simulink model "station_no_recovery"  (R2015a)
settings: Solver=ode45  StartTime=0  StopTime=5000  FixedStep=10  MaxStep=1  RelTol=1e-3
(part 3 of 4)

== system station_no_recovery/Восстанавливаемые объекты/САТУРН/Subsystem2 ==
  λ1 : Inport
  λ2 : Inport  Port=2
  M : Inport  Port=3
  dP : Inport  Port=4
  Pz : Inport  Port=5
  dt : Inport  Port=6
  trec : Inport  Port=7
  t_start : Inport  Port=8
  Chart : Stateflow chart  TreatAsAtomicUnit=on
  Clock : Clock
  Data Store Memory : DataStoreMemory  DataStoreName=t3_3
  Data Store Read : DataStoreRead  DataStoreName=t3_3
  Data Store Write : DataStoreWrite  DataStoreName=t3_3
  Element Exponential : Subsystem  mask(Element Exponential){}
      mask help:
      | <p>Возвращает вероятность безотказной работы невосстанавливаемого элемента
      | по экспоненциальному закону распределения.</p>
      | <p>Экспоненциальное (или показательное) распределение — абсолютно непрерывное
      | распределение, моделирующее время между двумя последовательными свершениями
      | одного и того же события.</p>
      | <p>Экспоненциальное распределение используют при оценке надежности сложных
      | технических систем, не подверженных износу и старению и в случаях, когда
      | отказы объектов имеют случайный характер.</p>
      mask Help:
      | <p>Возвращает вероятность безотказной работы невосстанавливаемого элемента по экспоненциальному
      | закону распределения.</p>
      | <p>Экспоненциальное распределение используют при оценке надежности сложных
      | технических систем, не подверженных износу и старению и в случаях, когда
      | отказы объектов имеют случайный характер.</p>
      | <p>Входной параметр λ - интенсивность событий в рассматриваемом потоке.</p>
      | <p>Выходной параметр P(t) - вероятность безотказной работы элемента.</p>
      mask Display:
      | image('images/png/exp.png')
      | port_label('input', 1, 'λ')
      | port_label('output', 1, 'P(t)')
  Element Normal : Subsystem  mask(Element Normal){}
      mask help:
      | <p>Возвращает вероятность безотказной работы невосстанавливаемого
      | элемента по нормальному закону распределения.</p>
      | <p>Нормальное распределение, также называемое распределением Гаусса или
      | Гаусса — Лапласа — распределение вероятностей, которое в одномерном
      | случае задаётся функцией плотности вероятности, совпадающей с функцией
      | Гаусса.</p>
      | <p>Нормальное распределение обычно используют при оценке надежности объектов,
      | основной причиной отказа которых является износ.</p>
      mask Help:
      | <p>Возвращает вероятность безотказной работы невосстанавливаемого
      | элемента по нормальному закону распределения.</p>
      | <p>Нормальное распределение обычно используют при оценке надежности объектов,
      | основной причиной отказа которых является износ.</p>
      | <p>Входные параметры:</p>
      | <p>λ - среднее квадратическое отклонение наработки до отказа,</p>
      | <p>М - математическое ожидание наработки до отказа.</p>
      | <p>Выходной параметр P(t) - вероятность безотказной работы элемента.</p>
      mask Display:
      | image('images/png/normal_nogrid.png')
      | port_label('input', 1, 'λ')
      | port_label('input', 2, 'M')
      | port_label('output', 1, 'P(t)')
  Сircuit Series : Subsystem  mask(Сircuit Series){}
      mask help:
      | <p>Возвращает вероятность безотказной работы двух последовательно соединенных
      | элементов.</p>
      | <p>В системе с последовательной структурой отказ любого компонента приводит
      | к отказу системы в целом.</p>
      mask Help:
      | <p>Возвращает вероятность безотказной работы двух последовательно соединенных
      | элементов.</p>
      | <p>Входные параметры:</p>
      | <p>P1 - вероятность безотказной работы первого элемента,</p>
      | <p>P2 - вероятность безотказной работы второго элемента.</p>
      | <p>Выходной параметр P12 - вероятность безотказной работы двух последовательно
      | соединенных элементов.</p>
      mask Display:
      | image('images/png/series2.png')
      | port_label('input', 1, 'P1')
      | port_label('input', 2, 'P2')
      | port_label('output', 1, 'P12')
  P : Outport
  wires:
  Element Exponential/1(P(t)1) -> Сircuit Series/1(P1)
  Element Normal/1(P(t)) -> Сircuit Series/2(P2)
  Chart/2(P) -> P/1
  λ2/1 -> Element Normal/1("lambda ")
  Clock/1 -> Chart/6(t)
  Сircuit Series/1(P12) -> Chart/7(P0)
  dt/1 -> Chart/2(delta_t)
  λ1/1 -> Element Exponential/1("lambda ")
  Pz/1 -> Chart/3(Pz)
  dP/1 -> Chart/5(dP)
  M/1 -> Element Normal/2("M ")
  trec/1 -> Chart/4(trec)
  Data Store Read/1 -> Element Exponential/2(t), Element Normal/3(t)
  Chart/1(tv) -> Data Store Write/1
  t_start/1 -> Chart/1(t_start)

== system station_no_recovery/Восстанавливаемые объекты/САТУРН/Subsystem3 ==
  λ1 : Inport
  λ2 : Inport  Port=2
  M : Inport  Port=3
  dP : Inport  Port=4
  Pz : Inport  Port=5
  dt : Inport  Port=6
  trec : Inport  Port=7
  t_start : Inport  Port=8
  Chart : Stateflow chart  TreatAsAtomicUnit=on
  Clock : Clock
  Data Store Memory : DataStoreMemory  DataStoreName=t3_4
  Data Store Read : DataStoreRead  DataStoreName=t3_4
  Data Store Write : DataStoreWrite  DataStoreName=t3_4
  Element Exponential : Subsystem  mask(Element Exponential){}
      mask help:
      | <p>Возвращает вероятность безотказной работы невосстанавливаемого элемента
      | по экспоненциальному закону распределения.</p>
      | <p>Экспоненциальное (или показательное) распределение — абсолютно непрерывное
      | распределение, моделирующее время между двумя последовательными свершениями
      | одного и того же события.</p>
      | <p>Экспоненциальное распределение используют при оценке надежности сложных
      | технических систем, не подверженных износу и старению и в случаях, когда
      | отказы объектов имеют случайный характер.</p>
      mask Help:
      | <p>Возвращает вероятность безотказной работы невосстанавливаемого элемента по экспоненциальному
      | закону распределения.</p>
      | <p>Экспоненциальное распределение используют при оценке надежности сложных
      | технических систем, не подверженных износу и старению и в случаях, когда
      | отказы объектов имеют случайный характер.</p>
      | <p>Входной параметр λ - интенсивность событий в рассматриваемом потоке.</p>
      | <p>Выходной параметр P(t) - вероятность безотказной работы элемента.</p>
      mask Display:
      | image('images/png/exp.png')
      | port_label('input', 1, 'λ')
      | port_label('output', 1, 'P(t)')
  Element Normal : Subsystem  mask(Element Normal){}
      mask help:
      | <p>Возвращает вероятность безотказной работы невосстанавливаемого
      | элемента по нормальному закону распределения.</p>
      | <p>Нормальное распределение, также называемое распределением Гаусса или
      | Гаусса — Лапласа — распределение вероятностей, которое в одномерном
      | случае задаётся функцией плотности вероятности, совпадающей с функцией
      | Гаусса.</p>
      | <p>Нормальное распределение обычно используют при оценке надежности объектов,
      | основной причиной отказа которых является износ.</p>
      mask Help:
      | <p>Возвращает вероятность безотказной работы невосстанавливаемого
      | элемента по нормальному закону распределения.</p>
      | <p>Нормальное распределение обычно используют при оценке надежности объектов,
      | основной причиной отказа которых является износ.</p>
      | <p>Входные параметры:</p>
      | <p>λ - среднее квадратическое отклонение наработки до отказа,</p>
      | <p>М - математическое ожидание наработки до отказа.</p>
      | <p>Выходной параметр P(t) - вероятность безотказной работы элемента.</p>
      mask Display:
      | image('images/png/normal_nogrid.png')
      | port_label('input', 1, 'λ')
      | port_label('input', 2, 'M')
      | port_label('output', 1, 'P(t)')
  Сircuit Series : Subsystem  mask(Сircuit Series){}
      mask help:
      | <p>Возвращает вероятность безотказной работы двух последовательно соединенных
      | элементов.</p>
      | <p>В системе с последовательной структурой отказ любого компонента приводит
      | к отказу системы в целом.</p>
      mask Help:
      | <p>Возвращает вероятность безотказной работы двух последовательно соединенных
      | элементов.</p>
      | <p>Входные параметры:</p>
      | <p>P1 - вероятность безотказной работы первого элемента,</p>
      | <p>P2 - вероятность безотказной работы второго элемента.</p>
      | <p>Выходной параметр P12 - вероятность безотказной работы двух последовательно
      | соединенных элементов.</p>
      mask Display:
      | image('images/png/series2.png')
      | port_label('input', 1, 'P1')
      | port_label('input', 2, 'P2')
      | port_label('output', 1, 'P12')
  P : Outport
  wires:
  t_start/1 -> Chart/1(t_start)
  Chart/1(tv) -> Data Store Write/1
  Data Store Read/1 -> Element Normal/3(t), Element Exponential/2(t)
  trec/1 -> Chart/4(trec)
  M/1 -> Element Normal/2("M ")
  dP/1 -> Chart/5(dP)
  Pz/1 -> Chart/3(Pz)
  λ1/1 -> Element Exponential/1("lambda ")
  dt/1 -> Chart/2(delta_t)
  Сircuit Series/1(P12) -> Chart/7(P0)
  Clock/1 -> Chart/6(t)
  λ2/1 -> Element Normal/1("lambda ")
  Chart/2(P) -> P/1
  Element Normal/1(P(t)) -> Сircuit Series/2(P2)
  Element Exponential/1(P(t)1) -> Сircuit Series/1(P1)

== system station_no_recovery/Восстанавливаемые объекты/САТУРН/Subsystem4 ==
  λ1 : Inport
  λ2 : Inport  Port=2
  M : Inport  Port=3
  dP : Inport  Port=4
  Pz : Inport  Port=5
  dt : Inport  Port=6
  trec : Inport  Port=7
  t_start : Inport  Port=8
  Chart : Stateflow chart  TreatAsAtomicUnit=on
  Clock : Clock
  Data Store Memory : DataStoreMemory  DataStoreName=t3_1
  Data Store Read : DataStoreRead  DataStoreName=t3_1
  Data Store Write : DataStoreWrite  DataStoreName=t3_1
  Element Exponential : Subsystem  mask(Element Exponential){}
      mask help:
      | <p>Возвращает вероятность безотказной работы невосстанавливаемого элемента
      | по экспоненциальному закону распределения.</p>
      | <p>Экспоненциальное (или показательное) распределение — абсолютно непрерывное
      | распределение, моделирующее время между двумя последовательными свершениями
      | одного и того же события.</p>
      | <p>Экспоненциальное распределение используют при оценке надежности сложных
      | технических систем, не подверженных износу и старению и в случаях, когда
      | отказы объектов имеют случайный характер.</p>
      mask Help:
      | <p>Возвращает вероятность безотказной работы невосстанавливаемого элемента по экспоненциальному
      | закону распределения.</p>
      | <p>Экспоненциальное распределение используют при оценке надежности сложных
      | технических систем, не подверженных износу и старению и в случаях, когда
      | отказы объектов имеют случайный характер.</p>
      | <p>Входной параметр λ - интенсивность событий в рассматриваемом потоке.</p>
      | <p>Выходной параметр P(t) - вероятность безотказной работы элемента.</p>
      mask Display:
      | image('images/png/exp.png')
      | port_label('input', 1, 'λ')
      | port_label('output', 1, 'P(t)')
  Element Normal : Subsystem  mask(Element Normal){}
      mask help:
      | <p>Возвращает вероятность безотказной работы невосстанавливаемого
      | элемента по нормальному закону распределения.</p>
      | <p>Нормальное распределение, также называемое распределением Гаусса или
      | Гаусса — Лапласа — распределение вероятностей, которое в одномерном
      | случае задаётся функцией плотности вероятности, совпадающей с функцией
      | Гаусса.</p>
      | <p>Нормальное распределение обычно используют при оценке надежности объектов,
      | основной причиной отказа которых является износ.</p>
      mask Help:
      | <p>Возвращает вероятность безотказной работы невосстанавливаемого
      | элемента по нормальному закону распределения.</p>
      | <p>Нормальное распределение обычно используют при оценке надежности объектов,
      | основной причиной отказа которых является износ.</p>
      | <p>Входные параметры:</p>
      | <p>λ - среднее квадратическое отклонение наработки до отказа,</p>
      | <p>М - математическое ожидание наработки до отказа.</p>
      | <p>Выходной параметр P(t) - вероятность безотказной работы элемента.</p>
      mask Display:
      | image('images/png/normal_nogrid.png')
      | port_label('input', 1, 'λ')
      | port_label('input', 2, 'M')
      | port_label('output', 1, 'P(t)')
  Сircuit Series : Subsystem  mask(Сircuit Series){}
      mask help:
      | <p>Возвращает вероятность безотказной работы двух последовательно соединенных
      | элементов.</p>
      | <p>В системе с последовательной структурой отказ любого компонента приводит
      | к отказу системы в целом.</p>
      mask Help:
      | <p>Возвращает вероятность безотказной работы двух последовательно соединенных
      | элементов.</p>
      | <p>Входные параметры:</p>
      | <p>P1 - вероятность безотказной работы первого элемента,</p>
      | <p>P2 - вероятность безотказной работы второго элемента.</p>
      | <p>Выходной параметр P12 - вероятность безотказной работы двух последовательно
      | соединенных элементов.</p>
      mask Display:
      | image('images/png/series2.png')
      | port_label('input', 1, 'P1')
      | port_label('input', 2, 'P2')
      | port_label('output', 1, 'P12')
  P : Outport
  wires:
  Element Exponential/1(P(t)1) -> Сircuit Series/1(P1)
  Element Normal/1(P(t)) -> Сircuit Series/2(P2)
  Chart/2(P) -> P/1
  λ2/1 -> Element Normal/1("lambda ")
  Clock/1 -> Chart/6(t)
  Сircuit Series/1(P12) -> Chart/7(P0)
  dt/1 -> Chart/2(delta_t)
  λ1/1 -> Element Exponential/1("lambda ")
  Pz/1 -> Chart/3(Pz)
  dP/1 -> Chart/5(dP)
  M/1 -> Element Normal/2("M ")
  trec/1 -> Chart/4(trec)
  Data Store Read/1 -> Element Exponential/2(t), Element Normal/3(t)
  Chart/1(tv) -> Data Store Write/1
  t_start/1 -> Chart/1(t_start)

== system station_no_recovery/Восстанавливаемые объекты/УРАЛ-6000/Subsystem1 ==
  λ1 : Inport
  λ2 : Inport  Port=2
  M : Inport  Port=3
  dP : Inport  Port=4
  Pz : Inport  Port=5
  dt : Inport  Port=6
  trec : Inport  Port=7
  t_start : Inport  Port=8
  Chart : Stateflow chart  TreatAsAtomicUnit=on
  Clock : Clock
  Data Store Memory : DataStoreMemory  DataStoreName=t2_2
  Data Store Read : DataStoreRead  DataStoreName=t2_2
  Data Store Write : DataStoreWrite  DataStoreName=t2_2
  Display : Display
  Element Exponential : Subsystem  mask(Element Exponential){}
      mask help:
      | <p>Возвращает вероятность безотказной работы невосстанавливаемого элемента
      | по экспоненциальному закону распределения.</p>
      | <p>Экспоненциальное (или показательное) распределение — абсолютно непрерывное
      | распределение, моделирующее время между двумя последовательными свершениями
      | одного и того же события.</p>
      | <p>Экспоненциальное распределение используют при оценке надежности сложных
      | технических систем, не подверженных износу и старению и в случаях, когда
      | отказы объектов имеют случайный характер.</p>
      mask Help:
      | <p>Возвращает вероятность безотказной работы невосстанавливаемого элемента по экспоненциальному
      | закону распределения.</p>
      | <p>Экспоненциальное распределение используют при оценке надежности сложных
      | технических систем, не подверженных износу и старению и в случаях, когда
      | отказы объектов имеют случайный характер.</p>
      | <p>Входной параметр λ - интенсивность событий в рассматриваемом потоке.</p>
      | <p>Выходной параметр P(t) - вероятность безотказной работы элемента.</p>
      mask Display:
      | image('images/png/exp.png')
      | port_label('input', 1, 'λ')
      | port_label('output', 1, 'P(t)')
  Element Normal : Subsystem  mask(Element Normal){}
      mask help:
      | <p>Возвращает вероятность безотказной работы невосстанавливаемого
      | элемента по нормальному закону распределения.</p>
      | <p>Нормальное распределение, также называемое распределением Гаусса или
      | Гаусса — Лапласа — распределение вероятностей, которое в одномерном
      | случае задаётся функцией плотности вероятности, совпадающей с функцией
      | Гаусса.</p>
      | <p>Нормальное распределение обычно используют при оценке надежности объектов,
      | основной причиной отказа которых является износ.</p>
      mask Help:
      | <p>Возвращает вероятность безотказной работы невосстанавливаемого
      | элемента по нормальному закону распределения.</p>
      | <p>Нормальное распределение обычно используют при оценке надежности объектов,
      | основной причиной отказа которых является износ.</p>
      | <p>Входные параметры:</p>
      | <p>λ - среднее квадратическое отклонение наработки до отказа,</p>
      | <p>М - математическое ожидание наработки до отказа.</p>
      | <p>Выходной параметр P(t) - вероятность безотказной работы элемента.</p>
      mask Display:
      | image('images/png/normal_nogrid.png')
      | port_label('input', 1, 'λ')
      | port_label('input', 2, 'M')
      | port_label('output', 1, 'P(t)')
  Mux : Mux  Inputs=2
  Сircuit Series : Subsystem  mask(Сircuit Series){}
      mask help:
      | <p>Возвращает вероятность безотказной работы двух последовательно соединенных
      | элементов.</p>
      | <p>В системе с последовательной структурой отказ любого компонента приводит
      | к отказу системы в целом.</p>
      mask Help:
      | <p>Возвращает вероятность безотказной работы двух последовательно соединенных
      | элементов.</p>
      | <p>Входные параметры:</p>
      | <p>P1 - вероятность безотказной работы первого элемента,</p>
      | <p>P2 - вероятность безотказной работы второго элемента.</p>
      | <p>Выходной параметр P12 - вероятность безотказной работы двух последовательно
      | соединенных элементов.</p>
      mask Display:
      | image('images/png/series2.png')
      | port_label('input', 1, 'P1')
      | port_label('input', 2, 'P2')
      | port_label('output', 1, 'P12')
  P : Outport
  wires:
  Data Store Read/1 -> Element Exponential/2(t), Mux/2, Element Normal/3(t)
  t_start/1 -> Chart/1(t_start)
  Chart/1(tv) -> Data Store Write/1
  Mux/1 -> Display/1
  Сircuit Series/1(P12) -> Chart/7(P0)
  trec/1 -> Chart/4(trec)
  M/1 -> Element Normal/2("M ")
  dP/1 -> Chart/5(dP)
  Pz/1 -> Chart/3(Pz)
  λ1/1 -> Element Exponential/1("lambda "), Mux/1
  dt/1 -> Chart/2(delta_t)
  Clock/1 -> Chart/6(t)
  λ2/1 -> Element Normal/1("lambda ")
  Chart/2(P) -> P/1
  Element Normal/1(P(t)) -> Сircuit Series/2(P2)
  Element Exponential/1(P(t)1) -> Сircuit Series/1(P1)

== system station_no_recovery/Восстанавливаемые объекты/УРАЛ-6000/Subsystem2 ==
  λ1 : Inport
  λ2 : Inport  Port=2
  M : Inport  Port=3
  dP : Inport  Port=4
  Pz : Inport  Port=5
  dt : Inport  Port=6
  trec : Inport  Port=7
  t_start : Inport  Port=8
  Chart : Stateflow chart  TreatAsAtomicUnit=on
  Clock : Clock
  Data Store Memory : DataStoreMemory  DataStoreName=t2_1
  Data Store Read : DataStoreRead  DataStoreName=t2_1
  Data Store Write : DataStoreWrite  DataStoreName=t2_1
  Display : Display
  Element Exponential : Subsystem  mask(Element Exponential){}
      mask help:
      | <p>Возвращает вероятность безотказной работы невосстанавливаемого элемента
      | по экспоненциальному закону распределения.</p>
      | <p>Экспоненциальное (или показательное) распределение — абсолютно непрерывное
      | распределение, моделирующее время между двумя последовательными свершениями
      | одного и того же события.</p>
      | <p>Экспоненциальное распределение используют при оценке надежности сложных
      | технических систем, не подверженных износу и старению и в случаях, когда
      | отказы объектов имеют случайный характер.</p>
      mask Help:
      | <p>Возвращает вероятность безотказной работы невосстанавливаемого элемента по экспоненциальному
      | закону распределения.</p>
      | <p>Экспоненциальное распределение используют при оценке надежности сложных
      | технических систем, не подверженных износу и старению и в случаях, когда
      | отказы объектов имеют случайный характер.</p>
      | <p>Входной параметр λ - интенсивность событий в рассматриваемом потоке.</p>
      | <p>Выходной параметр P(t) - вероятность безотказной работы элемента.</p>
      mask Display:
      | image('images/png/exp.png')
      | port_label('input', 1, 'λ')
      | port_label('output', 1, 'P(t)')
  Element Normal : Subsystem  mask(Element Normal){}
      mask help:
      | <p>Возвращает вероятность безотказной работы невосстанавливаемого
      | элемента по нормальному закону распределения.</p>
      | <p>Нормальное распределение, также называемое распределением Гаусса или
      | Гаусса — Лапласа — распределение вероятностей, которое в одномерном
      | случае задаётся функцией плотности вероятности, совпадающей с функцией
      | Гаусса.</p>
      | <p>Нормальное распределение обычно используют при оценке надежности объектов,
      | основной причиной отказа которых является износ.</p>
      mask Help:
      | <p>Возвращает вероятность безотказной работы невосстанавливаемого
      | элемента по нормальному закону распределения.</p>
      | <p>Нормальное распределение обычно используют при оценке надежности объектов,
      | основной причиной отказа которых является износ.</p>
      | <p>Входные параметры:</p>
      | <p>λ - среднее квадратическое отклонение наработки до отказа,</p>
      | <p>М - математическое ожидание наработки до отказа.</p>
      | <p>Выходной параметр P(t) - вероятность безотказной работы элемента.</p>
      mask Display:
      | image('images/png/normal_nogrid.png')
      | port_label('input', 1, 'λ')
      | port_label('input', 2, 'M')
      | port_label('output', 1, 'P(t)')
  Mux : Mux  Inputs=2
  Сircuit Series : Subsystem  mask(Сircuit Series){}
      mask help:
      | <p>Возвращает вероятность безотказной работы двух последовательно соединенных
      | элементов.</p>
      | <p>В системе с последовательной структурой отказ любого компонента приводит
      | к отказу системы в целом.</p>
      mask Help:
      | <p>Возвращает вероятность безотказной работы двух последовательно соединенных
      | элементов.</p>
      | <p>Входные параметры:</p>
      | <p>P1 - вероятность безотказной работы первого элемента,</p>
      | <p>P2 - вероятность безотказной работы второго элемента.</p>
      | <p>Выходной параметр P12 - вероятность безотказной работы двух последовательно
      | соединенных элементов.</p>
      mask Display:
      | image('images/png/series2.png')
      | port_label('input', 1, 'P1')
      | port_label('input', 2, 'P2')
      | port_label('output', 1, 'P12')
  P : Outport
  wires:
  Element Exponential/1(P(t)1) -> Сircuit Series/1(P1)
  Element Normal/1(P(t)) -> Сircuit Series/2(P2)
  Chart/2(P) -> P/1
  λ2/1 -> Element Normal/1("lambda ")
  Clock/1 -> Chart/6(t)
  dt/1 -> Chart/2(delta_t)
  λ1/1 -> Mux/1, Element Exponential/1("lambda ")
  Pz/1 -> Chart/3(Pz)
  dP/1 -> Chart/5(dP)
  M/1 -> Element Normal/2("M ")
  trec/1 -> Chart/4(trec)
  Сircuit Series/1(P12) -> Chart/7(P0)
  Mux/1 -> Display/1
  Chart/1(tv) -> Data Store Write/1
  t_start/1 -> Chart/1(t_start)
  Data Store Read/1 -> Element Normal/3(t), Mux/2, Element Exponential/2(t)

== system station_no_recovery/Восстанавливаемые объекты/УРАЛ-6000/Subsystem3 ==
  λ1 : Inport
  λ2 : Inport  Port=2
  M : Inport  Port=3
  dP : Inport  Port=4
  Pz : Inport  Port=5
  dt : Inport  Port=6
  trec : Inport  Port=7
  t_start : Inport  Port=8
  Chart : Stateflow chart  TreatAsAtomicUnit=on
  Clock : Clock
  Data Store Memory : DataStoreMemory  DataStoreName=t2_3
  Data Store Read : DataStoreRead  DataStoreName=t2_3
  Data Store Write : DataStoreWrite  DataStoreName=t2_3
  Display : Display
  Element Exponential : Subsystem  mask(Element Exponential){}
      mask help:
      | <p>Возвращает вероятность безотказной работы невосстанавливаемого элемента
      | по экспоненциальному закону распределения.</p>
      | <p>Экспоненциальное (или показательное) распределение — абсолютно непрерывное
      | распределение, моделирующее время между двумя последовательными свершениями
      | одного и того же события.</p>
      | <p>Экспоненциальное распределение используют при оценке надежности сложных
      | технических систем, не подверженных износу и старению и в случаях, когда
      | отказы объектов имеют случайный характер.</p>
      mask Help:
      | <p>Возвращает вероятность безотказной работы невосстанавливаемого элемента по экспоненциальному
      | закону распределения.</p>
      | <p>Экспоненциальное распределение используют при оценке надежности сложных
      | технических систем, не подверженных износу и старению и в случаях, когда
      | отказы объектов имеют случайный характер.</p>
      | <p>Входной параметр λ - интенсивность событий в рассматриваемом потоке.</p>
      | <p>Выходной параметр P(t) - вероятность безотказной работы элемента.</p>
      mask Display:
      | image('images/png/exp.png')
      | port_label('input', 1, 'λ')
      | port_label('output', 1, 'P(t)')
  Element Normal : Subsystem  mask(Element Normal){}
      mask help:
      | <p>Возвращает вероятность безотказной работы невосстанавливаемого
      | элемента по нормальному закону распределения.</p>
      | <p>Нормальное распределение, также называемое распределением Гаусса или
      | Гаусса — Лапласа — распределение вероятностей, которое в одномерном
      | случае задаётся функцией плотности вероятности, совпадающей с функцией
      | Гаусса.</p>
      | <p>Нормальное распределение обычно используют при оценке надежности объектов,
      | основной причиной отказа которых является износ.</p>
      mask Help:
      | <p>Возвращает вероятность безотказной работы невосстанавливаемого
      | элемента по нормальному закону распределения.</p>
      | <p>Нормальное распределение обычно используют при оценке надежности объектов,
      | основной причиной отказа которых является износ.</p>
      | <p>Входные параметры:</p>
      | <p>λ - среднее квадратическое отклонение наработки до отказа,</p>
      | <p>М - математическое ожидание наработки до отказа.</p>
      | <p>Выходной параметр P(t) - вероятность безотказной работы элемента.</p>
      mask Display:
      | image('images/png/normal_nogrid.png')
      | port_label('input', 1, 'λ')
      | port_label('input', 2, 'M')
      | port_label('output', 1, 'P(t)')
  Mux : Mux  Inputs=2
  Сircuit Series : Subsystem  mask(Сircuit Series){}
      mask help:
      | <p>Возвращает вероятность безотказной работы двух последовательно соединенных
      | элементов.</p>
      | <p>В системе с последовательной структурой отказ любого компонента приводит
      | к отказу системы в целом.</p>
      mask Help:
      | <p>Возвращает вероятность безотказной работы двух последовательно соединенных
      | элементов.</p>
      | <p>Входные параметры:</p>
      | <p>P1 - вероятность безотказной работы первого элемента,</p>
      | <p>P2 - вероятность безотказной работы второго элемента.</p>
      | <p>Выходной параметр P12 - вероятность безотказной работы двух последовательно
      | соединенных элементов.</p>
      mask Display:
      | image('images/png/series2.png')
      | port_label('input', 1, 'P1')
      | port_label('input', 2, 'P2')
      | port_label('output', 1, 'P12')
  P : Outport
  wires:
  Element Exponential/1(P(t)1) -> Сircuit Series/1(P1)
  Element Normal/1(P(t)) -> Сircuit Series/2(P2)
  Chart/2(P) -> P/1
  λ2/1 -> Element Normal/1("lambda ")
  Clock/1 -> Chart/6(t)
  dt/1 -> Chart/2(delta_t)
  λ1/1 -> Mux/1, Element Exponential/1("lambda ")
  Pz/1 -> Chart/3(Pz)
  dP/1 -> Chart/5(dP)
  M/1 -> Element Normal/2("M ")
  trec/1 -> Chart/4(trec)
  Сircuit Series/1(P12) -> Chart/7(P0)
  Mux/1 -> Display/1
  Chart/1(tv) -> Data Store Write/1
  t_start/1 -> Chart/1(t_start)
  Data Store Read/1 -> Element Normal/3(t), Mux/2, Element Exponential/2(t)

== system station_no_recovery/Восстанавливаемые объекты/УРАЛ-6000/Subsystem4 ==
  λ1 : Inport
  λ2 : Inport  Port=2
  M : Inport  Port=3
  dP : Inport  Port=4
  Pz : Inport  Port=5
  dt : Inport  Port=6
  trec : Inport  Port=7
  t_start : Inport  Port=8
  Chart : Stateflow chart  TreatAsAtomicUnit=on
  Clock : Clock
  Data Store Memory : DataStoreMemory  DataStoreName=t2_4
  Data Store Read : DataStoreRead  DataStoreName=t2_4
  Data Store Write : DataStoreWrite  DataStoreName=t2_4
  Display : Display
  Element Exponential : Subsystem  mask(Element Exponential){}
      mask help:
      | <p>Возвращает вероятность безотказной работы невосстанавливаемого элемента
      | по экспоненциальному закону распределения.</p>
      | <p>Экспоненциальное (или показательное) распределение — абсолютно непрерывное
      | распределение, моделирующее время между двумя последовательными свершениями
      | одного и того же события.</p>
      | <p>Экспоненциальное распределение используют при оценке надежности сложных
      | технических систем, не подверженных износу и старению и в случаях, когда
      | отказы объектов имеют случайный характер.</p>
      mask Help:
      | <p>Возвращает вероятность безотказной работы невосстанавливаемого элемента по экспоненциальному
      | закону распределения.</p>
      | <p>Экспоненциальное распределение используют при оценке надежности сложных
      | технических систем, не подверженных износу и старению и в случаях, когда
      | отказы объектов имеют случайный характер.</p>
      | <p>Входной параметр λ - интенсивность событий в рассматриваемом потоке.</p>
      | <p>Выходной параметр P(t) - вероятность безотказной работы элемента.</p>
      mask Display:
      | image('images/png/exp.png')
      | port_label('input', 1, 'λ')
      | port_label('output', 1, 'P(t)')
  Element Normal : Subsystem  mask(Element Normal){}
      mask help:
      | <p>Возвращает вероятность безотказной работы невосстанавливаемого
      | элемента по нормальному закону распределения.</p>
      | <p>Нормальное распределение, также называемое распределением Гаусса или
      | Гаусса — Лапласа — распределение вероятностей, которое в одномерном
      | случае задаётся функцией плотности вероятности, совпадающей с функцией
      | Гаусса.</p>
      | <p>Нормальное распределение обычно используют при оценке надежности объектов,
      | основной причиной отказа которых является износ.</p>
      mask Help:
      | <p>Возвращает вероятность безотказной работы невосстанавливаемого
      | элемента по нормальному закону распределения.</p>
      | <p>Нормальное распределение обычно используют при оценке надежности объектов,
      | основной причиной отказа которых является износ.</p>
      | <p>Входные параметры:</p>
      | <p>λ - среднее квадратическое отклонение наработки до отказа,</p>
      | <p>М - математическое ожидание наработки до отказа.</p>
      | <p>Выходной параметр P(t) - вероятность безотказной работы элемента.</p>
      mask Display:
      | image('images/png/normal_nogrid.png')
      | port_label('input', 1, 'λ')
      | port_label('input', 2, 'M')
      | port_label('output', 1, 'P(t)')
  Mux : Mux  Inputs=2
  Сircuit Series : Subsystem  mask(Сircuit Series){}
      mask help:
      | <p>Возвращает вероятность безотказной работы двух последовательно соединенных
      | элементов.</p>
      | <p>В системе с последовательной структурой отказ любого компонента приводит
      | к отказу системы в целом.</p>
      mask Help:
      | <p>Возвращает вероятность безотказной работы двух последовательно соединенных
      | элементов.</p>
      | <p>Входные параметры:</p>
      | <p>P1 - вероятность безотказной работы первого элемента,</p>
      | <p>P2 - вероятность безотказной работы второго элемента.</p>
      | <p>Выходной параметр P12 - вероятность безотказной работы двух последовательно
      | соединенных элементов.</p>
      mask Display:
      | image('images/png/series2.png')
      | port_label('input', 1, 'P1')
      | port_label('input', 2, 'P2')
      | port_label('output', 1, 'P12')
  P : Outport
  wires:
  Data Store Read/1 -> Element Exponential/2(t), Mux/2, Element Normal/3(t)
  t_start/1 -> Chart/1(t_start)
  Chart/1(tv) -> Data Store Write/1
  Mux/1 -> Display/1
  Сircuit Series/1(P12) -> Chart/7(P0)
  trec/1 -> Chart/4(trec)
  M/1 -> Element Normal/2("M ")
  dP/1 -> Chart/5(dP)
  Pz/1 -> Chart/3(Pz)
  λ1/1 -> Element Exponential/1("lambda "), Mux/1
  dt/1 -> Chart/2(delta_t)
  Clock/1 -> Chart/6(t)
  λ2/1 -> Element Normal/1("lambda ")
  Chart/2(P) -> P/1
  Element Normal/1(P(t)) -> Сircuit Series/2(P2)
  Element Exponential/1(P(t)1) -> Сircuit Series/1(P1)

== system station_no_recovery/Восстанавливаемые объекты/ЭГ-12/Subsystem1 ==
  λ1 : Inport
  λ2 : Inport  Port=2
  M : Inport  Port=3
  dP : Inport  Port=4
  Pz : Inport  Port=5
  dt : Inport  Port=6
  trec : Inport  Port=7
  t_start : Inport  Port=8
  Chart : Stateflow chart  TreatAsAtomicUnit=on
  Clock : Clock
  Data Store Memory : DataStoreMemory  DataStoreName=t5_2
  Data Store Read : DataStoreRead  DataStoreName=t5_2
  Data Store Write : DataStoreWrite  DataStoreName=t5_2
  Element Exponential : Subsystem  mask(Element Exponential){}
      mask help:
      | <p>Возвращает вероятность безотказной работы невосстанавливаемого элемента
      | по экспоненциальному закону распределения.</p>
      | <p>Экспоненциальное (или показательное) распределение — абсолютно непрерывное
      | распределение, моделирующее время между двумя последовательными свершениями
      | одного и того же события.</p>
      | <p>Экспоненциальное распределение используют при оценке надежности сложных
      | технических систем, не подверженных износу и старению и в случаях, когда
      | отказы объектов имеют случайный характер.</p>
      mask Help:
      | <p>Возвращает вероятность безотказной работы невосстанавливаемого элемента по экспоненциальному
      | закону распределения.</p>
      | <p>Экспоненциальное распределение используют при оценке надежности сложных
      | технических систем, не подверженных износу и старению и в случаях, когда
      | отказы объектов имеют случайный характер.</p>
      | <p>Входной параметр λ - интенсивность событий в рассматриваемом потоке.</p>
      | <p>Выходной параметр P(t) - вероятность безотказной работы элемента.</p>
      mask Display:
      | image('images/png/exp.png')
      | port_label('input', 1, 'λ')
      | port_label('output', 1, 'P(t)')
  Element Normal : Subsystem  mask(Element Normal){}
      mask help:
      | <p>Возвращает вероятность безотказной работы невосстанавливаемого
      | элемента по нормальному закону распределения.</p>
      | <p>Нормальное распределение, также называемое распределением Гаусса или
      | Гаусса — Лапласа — распределение вероятностей, которое в одномерном
      | случае задаётся функцией плотности вероятности, совпадающей с функцией
      | Гаусса.</p>
      | <p>Нормальное распределение обычно используют при оценке надежности объектов,
      | основной причиной отказа которых является износ.</p>
      mask Help:
      | <p>Возвращает вероятность безотказной работы невосстанавливаемого
      | элемента по нормальному закону распределения.</p>
      | <p>Нормальное распределение обычно используют при оценке надежности объектов,
      | основной причиной отказа которых является износ.</p>
      | <p>Входные параметры:</p>
      | <p>λ - среднее квадратическое отклонение наработки до отказа,</p>
      | <p>М - математическое ожидание наработки до отказа.</p>
      | <p>Выходной параметр P(t) - вероятность безотказной работы элемента.</p>
      mask Display:
      | image('images/png/normal_nogrid.png')
      | port_label('input', 1, 'λ')
      | port_label('input', 2, 'M')
      | port_label('output', 1, 'P(t)')
  Сircuit Series : Subsystem  mask(Сircuit Series){}
      mask help:
      | <p>Возвращает вероятность безотказной работы двух последовательно соединенных
      | элементов.</p>
      | <p>В системе с последовательной структурой отказ любого компонента приводит
      | к отказу системы в целом.</p>
      mask Help:
      | <p>Возвращает вероятность безотказной работы двух последовательно соединенных
      | элементов.</p>
      | <p>Входные параметры:</p>
      | <p>P1 - вероятность безотказной работы первого элемента,</p>
      | <p>P2 - вероятность безотказной работы второго элемента.</p>
      | <p>Выходной параметр P12 - вероятность безотказной работы двух последовательно
      | соединенных элементов.</p>
      mask Display:
      | image('images/png/series2.png')
      | port_label('input', 1, 'P1')
      | port_label('input', 2, 'P2')
      | port_label('output', 1, 'P12')
  P : Outport
  wires:
  Data Store Read/1 -> Element Exponential/2(t), Element Normal/3(t)
  Chart/1(tv) -> Data Store Write/1
  t_start/1 -> Chart/1(t_start)
  trec/1 -> Chart/4(trec)
  Element Exponential/1(P(t)1) -> Сircuit Series/1(P1)
  Element Normal/1(P(t)) -> Сircuit Series/2(P2)
  Chart/2(P) -> P/1
  λ2/1 -> Element Normal/1("lambda ")
  Clock/1 -> Chart/6(t)
  Сircuit Series/1(P12) -> Chart/7(P0)
  dt/1 -> Chart/2(delta_t)
  λ1/1 -> Element Exponential/1("lambda ")
  Pz/1 -> Chart/3(Pz)
  dP/1 -> Chart/5(dP)
  M/1 -> Element Normal/2("M ")

== system station_no_recovery/Восстанавливаемые объекты/ЭГ-12/Subsystem3 ==
  λ1 : Inport
  λ2 : Inport  Port=2
  M : Inport  Port=3
  dP : Inport  Port=4
  Pz : Inport  Port=5
  dt : Inport  Port=6
  trec : Inport  Port=7
  t_start : Inport  Port=8
  Chart : Stateflow chart  TreatAsAtomicUnit=on
  Clock : Clock
  Data Store Memory : DataStoreMemory  DataStoreName=t5_1
  Data Store Read : DataStoreRead  DataStoreName=t5_1
  Data Store Write : DataStoreWrite  DataStoreName=t5_1
  Element Exponential : Subsystem  mask(Element Exponential){}
      mask help:
      | <p>Возвращает вероятность безотказной работы невосстанавливаемого элемента
      | по экспоненциальному закону распределения.</p>
      | <p>Экспоненциальное (или показательное) распределение — абсолютно непрерывное
      | распределение, моделирующее время между двумя последовательными свершениями
      | одного и того же события.</p>
      | <p>Экспоненциальное распределение используют при оценке надежности сложных
      | технических систем, не подверженных износу и старению и в случаях, когда
      | отказы объектов имеют случайный характер.</p>
      mask Help:
      | <p>Возвращает вероятность безотказной работы невосстанавливаемого элемента по экспоненциальному
      | закону распределения.</p>
      | <p>Экспоненциальное распределение используют при оценке надежности сложных
      | технических систем, не подверженных износу и старению и в случаях, когда
      | отказы объектов имеют случайный характер.</p>
      | <p>Входной параметр λ - интенсивность событий в рассматриваемом потоке.</p>
      | <p>Выходной параметр P(t) - вероятность безотказной работы элемента.</p>
      mask Display:
      | image('images/png/exp.png')
      | port_label('input', 1, 'λ')
      | port_label('output', 1, 'P(t)')
  Element Normal : Subsystem  mask(Element Normal){}
      mask help:
      | <p>Возвращает вероятность безотказной работы невосстанавливаемого
      | элемента по нормальному закону распределения.</p>
      | <p>Нормальное распределение, также называемое распределением Гаусса или
      | Гаусса — Лапласа — распределение вероятностей, которое в одномерном
      | случае задаётся функцией плотности вероятности, совпадающей с функцией
      | Гаусса.</p>
      | <p>Нормальное распределение обычно используют при оценке надежности объектов,
      | основной причиной отказа которых является износ.</p>
      mask Help:
      | <p>Возвращает вероятность безотказной работы невосстанавливаемого
      | элемента по нормальному закону распределения.</p>
      | <p>Нормальное распределение обычно используют при оценке надежности объектов,
      | основной причиной отказа которых является износ.</p>
      | <p>Входные параметры:</p>
      | <p>λ - среднее квадратическое отклонение наработки до отказа,</p>
      | <p>М - математическое ожидание наработки до отказа.</p>
      | <p>Выходной параметр P(t) - вероятность безотказной работы элемента.</p>
      mask Display:
      | image('images/png/normal_nogrid.png')
      | port_label('input', 1, 'λ')
      | port_label('input', 2, 'M')
      | port_label('output', 1, 'P(t)')
  Сircuit Series : Subsystem  mask(Сircuit Series){}
      mask help:
      | <p>Возвращает вероятность безотказной работы двух последовательно соединенных
      | элементов.</p>
      | <p>В системе с последовательной структурой отказ любого компонента приводит
      | к отказу системы в целом.</p>
      mask Help:
      | <p>Возвращает вероятность безотказной работы двух последовательно соединенных
      | элементов.</p>
      | <p>Входные параметры:</p>
      | <p>P1 - вероятность безотказной работы первого элемента,</p>
      | <p>P2 - вероятность безотказной работы второго элемента.</p>
      | <p>Выходной параметр P12 - вероятность безотказной работы двух последовательно
      | соединенных элементов.</p>
      mask Display:
      | image('images/png/series2.png')
      | port_label('input', 1, 'P1')
      | port_label('input', 2, 'P2')
      | port_label('output', 1, 'P12')
  P : Outport
  wires:
  M/1 -> Element Normal/2("M ")
  dP/1 -> Chart/5(dP)
  Pz/1 -> Chart/3(Pz)
  λ1/1 -> Element Exponential/1("lambda ")
  dt/1 -> Chart/2(delta_t)
  Сircuit Series/1(P12) -> Chart/7(P0)
  Clock/1 -> Chart/6(t)
  λ2/1 -> Element Normal/1("lambda ")
  Chart/2(P) -> P/1
  Element Normal/1(P(t)) -> Сircuit Series/2(P2)
  Element Exponential/1(P(t)1) -> Сircuit Series/1(P1)
  trec/1 -> Chart/4(trec)
  t_start/1 -> Chart/1(t_start)
  Chart/1(tv) -> Data Store Write/1
  Data Store Read/1 -> Element Normal/3(t), Element Exponential/2(t)

== system station_no_recovery/Схема/Сircuit Bridge2/parallel circuit 1-2 4-5 1-3-5 4-3-2 ==
  P : Inport
  n Parallel Function : MATLAB Function  TreatAsAtomicUnit=on
  Pn : Outport
  wires:
  P/1 -> n Parallel Function/1(P)
  n Parallel Function/1(Pn) -> Pn/1

== system station_no_recovery/Схема/Сircuit Bridge2/series circuit 1 - 2 ==
  P1 : Inport
  P2 : Inport  Port=2
  Fcn : Fcn  Expr=u(1)*u(2)
  Mux : Mux  Inputs=2
  P12 : Outport
  wires:
  Mux/1 -> Fcn/1
  P1/1 -> Mux/1
  Fcn/1 -> P12/1
  P2/1 -> Mux/2

== system station_no_recovery/Схема/Сircuit Bridge2/series circuit 1, 3, 5 ==
  P : Inport
  n Series Function : MATLAB Function  TreatAsAtomicUnit=on
  Pn : Outport
  wires:
  P/1 -> n Series Function/1(P)
  n Series Function/1(Pn) -> Pn/1

== system station_no_recovery/Схема/Сircuit Bridge2/series circuit 4 - 5 ==
  P1 : Inport
  P2 : Inport  Port=2
  Fcn : Fcn  Expr=u(1)*u(2)
  Mux : Mux  Inputs=2
  P12 : Outport
  wires:
  Mux/1 -> Fcn/1
  P1/1 -> Mux/1
  Fcn/1 -> P12/1
  P2/1 -> Mux/2

== system station_no_recovery/Схема/Сircuit Bridge2/series circuit 4, 3, 2 ==
  P : Inport
  n Series Function : MATLAB Function  TreatAsAtomicUnit=on
  Pn : Outport
  wires:
  P/1 -> n Series Function/1(P)
  n Series Function/1(Pn) -> Pn/1

== system station_no_recovery/Восстанавливаемые объекты/ГТЭ-6//6,3/Subsystem1/Element Exponential ==
  note: интенсивность событий
      | в рассматриваемом потоке
  "lambda " : Inport
  t : Inport  Port=2
  Divide : Product  Inputs=**
  Gain : Gain  Gain=-1
  Math Function : Math  SaturateOnIntegerOverflow=on
  P(t)1 : Outport
  wires:
  Divide/1 -> Gain/1
  t/1 -> Divide/1
  Gain/1 -> Math Function/1
  Math Function/1 -> P(t)1/1
  "lambda "/1 -> Divide/2

== system station_no_recovery/Восстанавливаемые объекты/ГТЭ-6//6,3/Subsystem1/Element Normal ==
  note: математическое ожидание
      | наработки до отказа
  note: среднее квадратическое
      | отклонение наработки
      | до отказа
  "lambda " : Inport
  "M " : Inport  Port=2
  t : Inport  Port=3
  1-Q(t)1 : Fcn  Expr=1-u(1)
  MATLAB Function : MATLAB Function  TreatAsAtomicUnit=on
  P(t) : Outport
  wires:
  t/1 -> MATLAB Function/1(t)
  MATLAB Function/1(y) -> 1-Q(t)1/1
  "lambda "/1 -> MATLAB Function/2(sigma)
  1-Q(t)1/1 -> P(t)/1
  "M "/1 -> MATLAB Function/3(M)

== system station_no_recovery/Восстанавливаемые объекты/ГТЭ-6//6,3/Subsystem1/Сircuit Series ==
  P1 : Inport
  P2 : Inport  Port=2
  Fcn : Fcn  Expr=u(1)*u(2)
  Mux : Mux  Inputs=2
  P12 : Outport
  wires:
  Mux/1 -> Fcn/1
  P1/1 -> Mux/1
  Fcn/1 -> P12/1
  P2/1 -> Mux/2

== system station_no_recovery/Восстанавливаемые объекты/ГТЭ-6//6,3/Subsystem2/Element Exponential ==
  note: интенсивность событий
      | в рассматриваемом потоке
  "lambda " : Inport
  t : Inport  Port=2
  Divide : Product  Inputs=**
  Gain : Gain  Gain=-1
  Math Function : Math  SaturateOnIntegerOverflow=on
  P(t)1 : Outport
  wires:
  "lambda "/1 -> Divide/2
  Math Function/1 -> P(t)1/1
  Gain/1 -> Math Function/1
  t/1 -> Divide/1
  Divide/1 -> Gain/1

== system station_no_recovery/Восстанавливаемые объекты/ГТЭ-6//6,3/Subsystem2/Element Normal ==
  note: среднее квадратическое
      | отклонение наработки
      | до отказа
  note: математическое ожидание
      | наработки до отказа
  "lambda " : Inport
  "M " : Inport  Port=2
  t : Inport  Port=3
  1-Q(t)1 : Fcn  Expr=1-u(1)
  MATLAB Function : MATLAB Function  TreatAsAtomicUnit=on
  P(t) : Outport
  wires:
  "M "/1 -> MATLAB Function/3(M)
  1-Q(t)1/1 -> P(t)/1
  "lambda "/1 -> MATLAB Function/2(sigma)
  MATLAB Function/1(y) -> 1-Q(t)1/1
  t/1 -> MATLAB Function/1(t)

== system station_no_recovery/Восстанавливаемые объекты/ГТЭ-6//6,3/Subsystem2/Сircuit Series ==
  P1 : Inport
  P2 : Inport  Port=2
  Fcn : Fcn  Expr=u(1)*u(2)
  Mux : Mux  Inputs=2
  P12 : Outport
  wires:
  P2/1 -> Mux/2
  Fcn/1 -> P12/1
  P1/1 -> Mux/1
  Mux/1 -> Fcn/1

== system station_no_recovery/Восстанавливаемые объекты/ПАЭС-2500/Subsystem/Element Exponential ==
  note: интенсивность событий
      | в рассматриваемом потоке
  "lambda " : Inport
  t : Inport  Port=2
  Divide : Product  Inputs=**
  Gain : Gain  Gain=-1
  Math Function : Math  SaturateOnIntegerOverflow=on
  P(t)1 : Outport
  wires:
  "lambda "/1 -> Divide/2
  Math Function/1 -> P(t)1/1
  Gain/1 -> Math Function/1
  t/1 -> Divide/1
  Divide/1 -> Gain/1

== system station_no_recovery/Восстанавливаемые объекты/ПАЭС-2500/Subsystem/Element Exponential1 ==
  note: интенсивность событий
      | в рассматриваемом потоке
  "lambda " : Inport
  t : Inport  Port=2
  Divide : Product  Inputs=**
  Gain : Gain  Gain=-1
  Math Function : Math  SaturateOnIntegerOverflow=on
  P(t)1 : Outport
  wires:
  Divide/1 -> Gain/1
  t/1 -> Divide/1
  Gain/1 -> Math Function/1
  Math Function/1 -> P(t)1/1
  "lambda "/1 -> Divide/2

== system station_no_recovery/Восстанавливаемые объекты/ПАЭС-2500/Subsystem/Element Normal ==
  note: среднее квадратическое
      | отклонение наработки
      | до отказа
  note: математическое ожидание
      | наработки до отказа
  "lambda " : Inport
  "M " : Inport  Port=2
  t : Inport  Port=3
  1-Q(t)1 : Fcn  Expr=1-u(1)
  MATLAB Function : MATLAB Function  TreatAsAtomicUnit=on
  P(t) : Outport
  wires:
  "M "/1 -> MATLAB Function/3(M)
  1-Q(t)1/1 -> P(t)/1
  "lambda "/1 -> MATLAB Function/2(sigma)
  MATLAB Function/1(y) -> 1-Q(t)1/1
  t/1 -> MATLAB Function/1(t)

== system station_no_recovery/Восстанавливаемые объекты/ПАЭС-2500/Subsystem/Element Normal1 ==
  note: математическое ожидание
      | наработки до отказа
  note: среднее квадратическое
      | отклонение наработки
      | до отказа
  "lambda " : Inport
  "M " : Inport  Port=2
  t : Inport  Port=3
  1-Q(t)1 : Fcn  Expr=1-u(1)
  MATLAB Function : MATLAB Function  TreatAsAtomicUnit=on
  P(t) : Outport
  wires:
  t/1 -> MATLAB Function/1(t)
  MATLAB Function/1(y) -> 1-Q(t)1/1
  "lambda "/1 -> MATLAB Function/2(sigma)
  1-Q(t)1/1 -> P(t)/1
  "M "/1 -> MATLAB Function/3(M)

== system station_no_recovery/Восстанавливаемые объекты/ПАЭС-2500/Subsystem/Сircuit Series ==
  P1 : Inport
  P2 : Inport  Port=2
  Fcn : Fcn  Expr=u(1)*u(2)
  Mux : Mux  Inputs=2
  P12 : Outport
  wires:
  P2/1 -> Mux/2
  Fcn/1 -> P12/1
  P1/1 -> Mux/1
  Mux/1 -> Fcn/1

== system station_no_recovery/Восстанавливаемые объекты/ПАЭС-2500/Subsystem/Сircuit Series1 ==
  P1 : Inport
  P2 : Inport  Port=2
  Fcn : Fcn  Expr=u(1)*u(2)
  Mux : Mux  Inputs=2
  P12 : Outport
  wires:
  Mux/1 -> Fcn/1
  P1/1 -> Mux/1
  Fcn/1 -> P12/1
  P2/1 -> Mux/2

== system station_no_recovery/Восстанавливаемые объекты/ПАЭС-2500/Subsystem1/Element Exponential ==
  note: интенсивность событий
      | в рассматриваемом потоке
  "lambda " : Inport
  t : Inport  Port=2
  Divide : Product  Inputs=**
  Gain : Gain  Gain=-1
  Math Function : Math  SaturateOnIntegerOverflow=on
  P(t)1 : Outport
  wires:
  Divide/1 -> Gain/1
  t/1 -> Divide/1
  Gain/1 -> Math Function/1
  Math Function/1 -> P(t)1/1
  "lambda "/1 -> Divide/2

== system station_no_recovery/Восстанавливаемые объекты/ПАЭС-2500/Subsystem1/Element Exponential1 ==
  note: интенсивность событий
      | в рассматриваемом потоке
  "lambda " : Inport
  t : Inport  Port=2
  Divide : Product  Inputs=**
  Gain : Gain  Gain=-1
  Math Function : Math  SaturateOnIntegerOverflow=on
  P(t)1 : Outport
  wires:
  "lambda "/1 -> Divide/2
  Math Function/1 -> P(t)1/1
  Gain/1 -> Math Function/1
  t/1 -> Divide/1
  Divide/1 -> Gain/1

== system station_no_recovery/Восстанавливаемые объекты/ПАЭС-2500/Subsystem1/Element Normal ==
  note: математическое ожидание
      | наработки до отказа
  note: среднее квадратическое
      | отклонение наработки
      | до отказа
  "lambda " : Inport
  "M " : Inport  Port=2
  t : Inport  Port=3
  1-Q(t)1 : Fcn  Expr=1-u(1)
  MATLAB Function : MATLAB Function  TreatAsAtomicUnit=on
  P(t) : Outport
  wires:
  t/1 -> MATLAB Function/1(t)
  MATLAB Function/1(y) -> 1-Q(t)1/1
  "lambda "/1 -> MATLAB Function/2(sigma)
  1-Q(t)1/1 -> P(t)/1
  "M "/1 -> MATLAB Function/3(M)

== system station_no_recovery/Восстанавливаемые объекты/ПАЭС-2500/Subsystem1/Element Normal1 ==
  note: среднее квадратическое
      | отклонение наработки
      | до отказа
  note: математическое ожидание
      | наработки до отказа
  "lambda " : Inport
  "M " : Inport  Port=2
  t : Inport  Port=3
  1-Q(t)1 : Fcn  Expr=1-u(1)
  MATLAB Function : MATLAB Function  TreatAsAtomicUnit=on
  P(t) : Outport
  wires:
  "M "/1 -> MATLAB Function/3(M)
  1-Q(t)1/1 -> P(t)/1
  "lambda "/1 -> MATLAB Function/2(sigma)
  MATLAB Function/1(y) -> 1-Q(t)1/1
  t/1 -> MATLAB Function/1(t)

== system station_no_recovery/Восстанавливаемые объекты/ПАЭС-2500/Subsystem1/Сircuit Series ==
  P1 : Inport
  P2 : Inport  Port=2
  Fcn : Fcn  Expr=u(1)*u(2)
  Mux : Mux  Inputs=2
  P12 : Outport
  wires:
  Mux/1 -> Fcn/1
  P1/1 -> Mux/1
  Fcn/1 -> P12/1
  P2/1 -> Mux/2

== system station_no_recovery/Восстанавливаемые объекты/ПАЭС-2500/Subsystem1/Сircuit Series1 ==
  P1 : Inport
  P2 : Inport  Port=2
  Fcn : Fcn  Expr=u(1)*u(2)
  Mux : Mux  Inputs=2
  P12 : Outport
  wires:
  P2/1 -> Mux/2
  Fcn/1 -> P12/1
  P1/1 -> Mux/1
  Mux/1 -> Fcn/1

== system station_no_recovery/Восстанавливаемые объекты/ПАЭС-2500/Subsystem2/Element Exponential ==
  note: интенсивность событий
      | в рассматриваемом потоке
  "lambda " : Inport
  t : Inport  Port=2
  Divide : Product  Inputs=**
  Gain : Gain  Gain=-1
  Math Function : Math  SaturateOnIntegerOverflow=on
  P(t)1 : Outport
  wires:
  Divide/1 -> Gain/1
  t/1 -> Divide/1
  Gain/1 -> Math Function/1
  Math Function/1 -> P(t)1/1
  "lambda "/1 -> Divide/2
